simulink model "plant"  (R2024a)
settings: Solver=VariableStepAuto  StartTime=0.0  StopTime=10.0  RelTol=1e-3
settings Model: Creator=mikom  LastModifiedBy=mikom

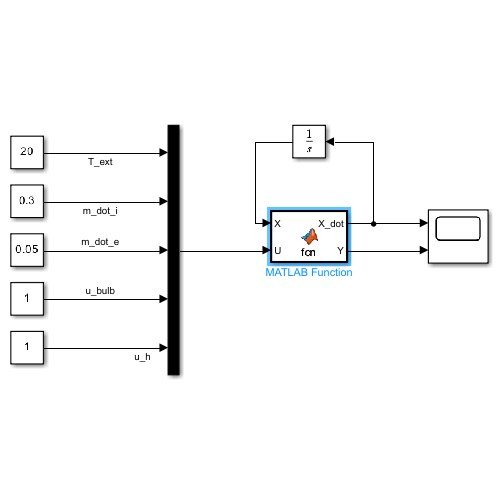
[thumbnail: Simulink's stored preview of the top-level diagram]
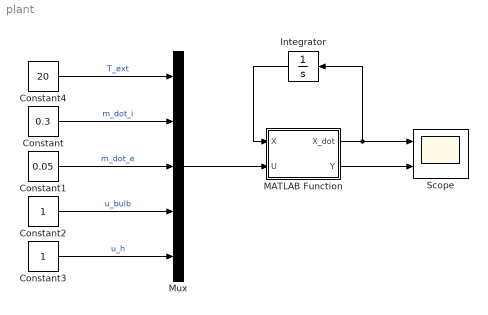
== system plant ==
  Constant : Constant  Value=0.3
  Constant1 : Constant  Value=0.05
  Constant2 : Constant
  Constant3 : Constant
  Constant4 : Constant  Value=20
  Integrator : Integrator  InitialCondition=[20;20;20]
  MATLAB Function : MATLAB Function  TreatAsAtomicUnit=on
  Mux : Mux  Inputs=5
  Scope : Scope  NumInputPorts=2
  wires:
  Mux/1 -> MATLAB Function/2(U)
  Constant/1 -> Mux/2  "m_dot_i"
  Constant1/1 -> Mux/3  "m_dot_e"
  Constant2/1 -> Mux/4  "u_bulb"
  Constant3/1 -> Mux/5  "u_h"
  MATLAB Function/2(Y) -> Scope/2
  MATLAB Function/1(X_dot) -> Scope/1, Integrator/1
  Integrator/1 -> MATLAB Function/1(X)
  Constant4/1 -> Mux/1  "T_ext"

== matlab function plant/MATLAB Function ==
  data: X input; X_dot output; U input; Y output
function [X_dot, Y]= fcn(X, U)
    %#codegen
    
    % Ensure Simulink knows the sizes
    X = X(:).'; % Ensure X is a row vector
    U = U(:).'; % Ensure U is a row vector

    % change this MANUALLY
    plant = ...
    @(in1,in2)deal([in1(:,1).*(-2.436795613767895e-2)+in1(:,3).*2.436795613767895e-2+in2(:,4).*1.827596710325921+((in2(:,3)+in2(:,2)).*(in1(:,2)-(in1(:,1).*in2(:,2).*1.005e+3+in1(:,3).*in2(:,3).*1.005e+3)./(in2(:,3).*1.005e+3+in2(:,2).*1.005e+3)).*1.020408163265306e+2)./(in2(:,3).*1.005e+3+in2(:,2).*1.005e+3+1.0),in1(:,3)./5.0e+1-in1(:,2)./5.0e+1+in2(:,5).*2.0-(in2(:,3)+in2(:,2)).*(in1(:,2)-(in1(:,1).*in2(:,2).*1.005e+3+in1(:,3).*in2(:,3).*1.005e+3)./(in2(:,3).*1.005e+3+in2(:,2).*1.005e+3)).*(2.01e+2./1.0e+1),in1(:,1)./1.0e+3-in1(:,3)./1.0e+3],[in1(:,1),(in1(:,1).*in2(:,2).*1.005e+3+in1(:,3).*in2(:,3).*1.005e+3)./(in2(:,3).*1.005e+3+in2(:,2).*1.005e+3),(in1(:,2)+in1(:,1).*in2(:,2).*1.005e+3+in1(:,3).*in2(:,3).*1.005e+3)./(in2(:,3).*1.005e+3+in2(:,2).*1.005e+3+1.0),in2(:,4).*2.0]);
    % <--- That one
    
    [a, b] = plant(X, U);
    X_dot = a(:); 
    Y = b(:);
end
